simulink model "Model"  (R2021b)
settings: Solver=FixedStepAuto  StartTime=0.0  StopTime=simulation_time  FixedStep=0.02  RelTol=1e-3
values from neighbouring files (symbols this model uses):
  Cfx = 0.08268    [QuadStateSpaceModel.m]
  controller_flag = 1    [Simulation.m]
  d = 0.21    [QuadStateSpaceModel.m]
  g = 9.81    [QuadStateSpaceModel.m]
  Ix = 0.01    [QuadStateSpaceModel.m]
  Iy = 0.01    [QuadStateSpaceModel.m]
  Iz = 0.02    [QuadStateSpaceModel.m]
  Khover = correction(Khover)    [QuadStateSpaceModel.m]
  m = 1    [QuadStateSpaceModel.m]
  rho = 1.1840    (= 1.184)    [QuadStateSpaceModel.m]
libraries: sharedtransform x2, uavutilslib x2, shared6dof x2, aerolibasang x2, slpidlib x1
settings Model: Creator=siaem  LastModifiedBy=siaem
settings SolverCC: AlgebraicLoopSolver=TrustRegion
settings DataIOCC: ReturnWorkspaceOutputs=off
settings OptimizationCC: DefaultParameterBehavior=Inlined  EnhancedBackFolding=on  PassReuseOutputArgsAs=Individual arguments  ZeroExternalMemoryAtStartup=off  ZeroInternalMemoryAtStartup=off  MaxStackSize=64  OptimizeBlockOrder=speed  DifferentSizesBufferReuse=on  OptimizationCustomize=off  EfficientTunableParamExpr=on
settings DebuggingCC: ParameterTunabilityLossMsg=error  SFMachineParentedDataDiag=warning  ArithmeticOperatorsInVariantConditions=warning
settings HardwareCC: ProdBitPerPointer=32  ProdBitPerSizeT=32  ProdBitPerPtrDiffT=32  ProdLargestAtomicFloat=None  ProdIntDivRoundTo=Undefined  ProdEndianess=Unspecified  ProdWordSize=32  ProdHWDeviceType=Generic->Unspecified (assume 32-bit Generic)
settings SFSimCC: MATLABDynamicMemAlloc=off  CustomCodeUndefinedFunction=UseInterfaceOnly
settings RTWCC: Description=Embedded Coder  SystemTargetFile=ert.tlc  TemplateMakefile=ert_default_tmf  Toolchain=Catkin
settings CodeAppCC: ForceParamTrailComments=on  IgnoreCustomStorageClasses=off  OperatorAnnotations=on  SimulinkDataObjDesc=on  SFDataObjDesc=on  InsertBlockDesc=on
settings ERTTargetCC: ERTCustomFileTemplate=example_file_process.tlc

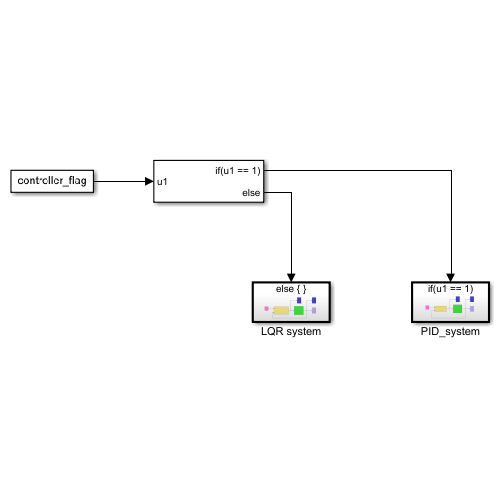
[thumbnail: Simulink's stored preview of the top-level diagram]
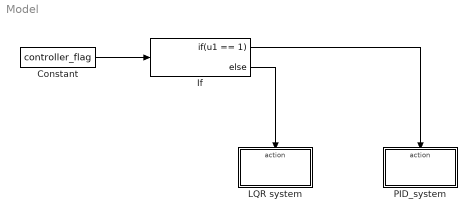
== system Model ==
  Constant : Constant  Value=controller_flag
  If : If  IfExpression=u1 == 1
  LQR system : Subsystem  TreatAsAtomicUnit=on
  PID_system : Subsystem  TreatAsAtomicUnit=on
  wires:
  Constant/1 -> If/1
  If/1 -> PID_system/Action
  If/2 -> LQR system/Action

== system Model/LQR system ==
  Action Port : ActionPort  ActionPortLabel=else
  Animation : Subsystem  Commented=on
  Controller : Subsystem
  Force & Moment Visualizer : Subsystem
  Setpoint : Subsystem
  States Visualizer : Subsystem
  quadrotor dynamic model : Subsystem
  wires:
  Controller/1(Forces/Moments) -> quadrotor dynamic model/1(Actuators), Force & Moment Visualizer/1(input)
  quadrotor dynamic model/1(States) -> Controller/2(States), Animation/1(In1), States Visualizer/1(output)
  Setpoint/1(Out1) -> Controller/1(setpoint)

== system Model/PID_system ==
  Action Port : ActionPort  ActionPortLabel=if(u1 == 1)
  Animation : Subsystem  Commented=on
  Controller : Subsystem
  Force & Moment Visualizer : Subsystem
  Setpoint : Subsystem
  States Visualizer : Subsystem
  quadrotor dynamic model : Subsystem
  wires:
  Setpoint/1(Out1) -> Controller/1(Setpoint)
  Controller/1(Forces Moments) -> quadrotor dynamic model/1(Actuators), Force & Moment Visualizer/1(input)
  quadrotor dynamic model/1(States) -> Animation/1(In1), States Visualizer/1(output), Controller/2(states)

== system Model/LQR system/Animation ==
  In1 : Inport
  Bus Selector : BusSelector  OutputSignals=X_e,attitude
  Rotation Angles to Quaternions : sharedtransform/Rotation Angles to Quaternions  rotationOrder=XYZ  aMode=aMode
      settings: SourceProductBaseCode=AE,PW,DR,MT,UV,VE
  UAV Animation : uavutilslib/UAV Animation  UAVType=Multirotor  UAVSize=1  InertialZDirection=Down  SampleTime=-1
      settings: SourceProductBaseCode=UV
  wires:
  Bus Selector/2 -> Rotation Angles to Quaternions/1  "<attitude>"
  Bus Selector/1 -> UAV Animation/1  "<X_e>"
  Rotation Angles to Quaternions/1 -> UAV Animation/2
  In1/1 -> Bus Selector/1

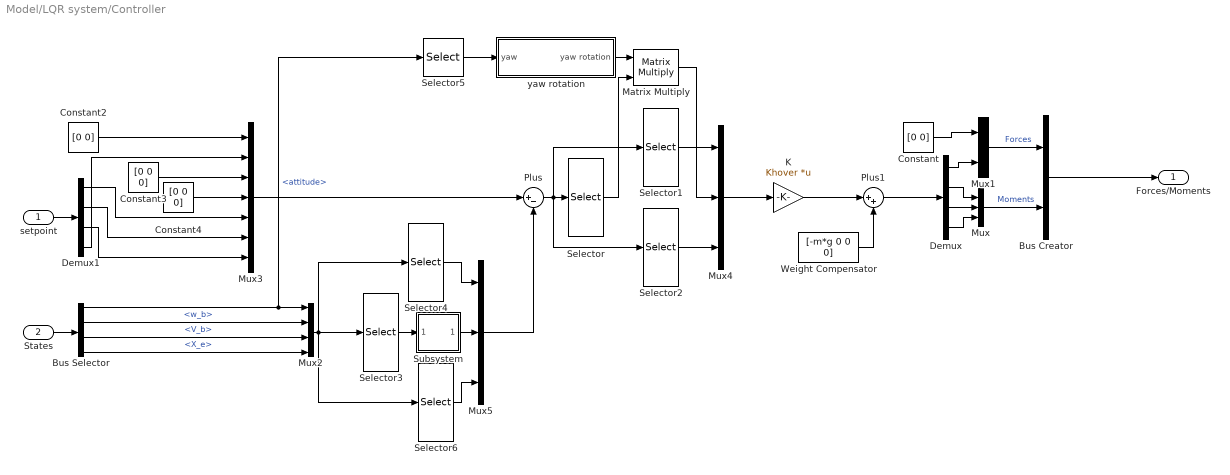
== system Model/LQR system/Controller ==
  setpoint : Inport
  States : Inport  Port=2
  Bus Creator : BusCreator  Inputs=2
  Bus Selector : BusSelector  OutputSignals=attitude,w_b,V_b,X_e
  Constant : Constant  Value=[0 0]
  Constant2 : Constant  Value=[0 0]
  Constant3 : Constant  Value=[0 0 0]
  Constant4 : Constant  Value=[0 0 0]
  Demux : Demux
  Demux1 : Demux
  K : Gain  Gain=Khover  Multiplication=Matrix(K*u) (u vector)
  Matrix Multiply : Product  Multiplication=Matrix(*)
  Mux : Mux  Inputs=3
  Mux1 : Mux  Inputs=2
  Mux2 : Mux
  Mux3 : Mux  Inputs=7
  Mux4 : Mux  Inputs=3
  Mux5 : Mux  Inputs=3
  Plus : Sum  Inputs=|+-
  Plus1 : Sum  Inputs=|++
  Selector : Selector  InputPortWidth=12  IndexOptions=Index vector (dialog)  Indices=[10 11]  OutputSizes=1
  Selector1 : Selector  InputPortWidth=12  IndexOptions=Index vector (dialog)  Indices=[1:9]  OutputSizes=1
  Selector2 : Selector  InputPortWidth=12  IndexOptions=Index vector (dialog)  Indices=12  OutputSizes=1
  Selector3 : Selector  InputPortWidth=12  IndexOptions=Index vector (dialog)  Indices=3  OutputSizes=1
  Selector4 : Selector  InputPortWidth=12  IndexOptions=Index vector (dialog)  Indices=[1,2]  OutputSizes=1
  Selector5 : Selector  InputPortWidth=3  IndexOptions=Index vector (dialog)  Indices=3  OutputSizes=1
  Selector6 : Selector  InputPortWidth=12  IndexOptions=Index vector (dialog)  Indices=[4:12]  OutputSizes=1
  Subsystem : Subsystem
  Weight Compensator : Constant  Value=[-m*g 0 0 0]
  yaw rotation : Subsystem
  Forces/Moments : Outport  VectorParamsAs1DForOutWhenUnconnected=off
  wires:
  Plus/1 -> Selector2/1, Selector1/1, Selector/1
  K/1 -> Plus1/1
  Weight Compensator/1 -> Plus1/2
  Plus1/1 -> Demux/1
  Demux/2 -> Mux/1
  Demux/3 -> Mux/2
  Demux/4 -> Mux/3
  Bus Creator/1 -> Forces/Moments/1
  Mux/1 -> Bus Creator/2  "Moments"
  Demux/1 -> Mux1/2
  Constant/1 -> Mux1/1
  Mux1/1 -> Bus Creator/1  "Forces"
  States/1 -> Bus Selector/1
  Bus Selector/1 -> Mux2/1, Selector5/1  "<attitude>"
  Bus Selector/2 -> Mux2/2  "<w_b>"
  Bus Selector/3 -> Mux2/3  "<V_b>"
  Bus Selector/4 -> Mux2/4  "<X_e>"
  setpoint/1 -> Demux1/1
  Demux1/4 -> Mux3/2
  Demux1/1 -> Mux3/5
  Demux1/2 -> Mux3/6
  Demux1/3 -> Mux3/7
  Constant2/1 -> Mux3/1
  Constant3/1 -> Mux3/3
  Constant4/1 -> Mux3/4
  Mux3/1 -> Plus/1
  Selector5/1 -> yaw rotation/1(yaw)
  yaw rotation/1(yaw rotation) -> Matrix Multiply/1
  Selector/1 -> Matrix Multiply/2
  Matrix Multiply/1 -> Mux4/2
  Selector1/1 -> Mux4/1
  Mux4/1 -> K/1
  Selector2/1 -> Mux4/3
  Mux2/1 -> Selector6/1, Selector4/1, Selector3/1
  Selector3/1 -> Subsystem/1(In1)
  Subsystem/1(Out1) -> Mux5/2
  Selector4/1 -> Mux5/1
  Selector6/1 -> Mux5/3
  Mux5/1 -> Plus/2

== system Model/LQR system/Force & Moment Visualizer ==
  input : Inport
  Demux3 : Demux
  Gain : Gain  Gain=-1
  Scope3 : Scope  NumInputPorts=4
  Selector : Selector  InputPortWidth=6  IndexOptions=Index vector (dialog)  Indices=[3, 4, 5, 6]  OutputSizes=1
  wires:
  Selector/1 -> Demux3/1
  Demux3/2 -> Scope3/2  "Tx"
  input/1 -> Selector/1
  Demux3/4 -> Scope3/4  "Tz"
  Demux3/3 -> Scope3/3  "Ty"
  Demux3/1 -> Gain/1  "Ft"
  Gain/1 -> Scope3/1

== system Model/LQR system/Setpoint ==
  From Workspace : FromWorkspace  VariableName=setpoint
  Out1 : Outport  VectorParamsAs1DForOutWhenUnconnected=off
  wires:
  From Workspace/1 -> Out1/1

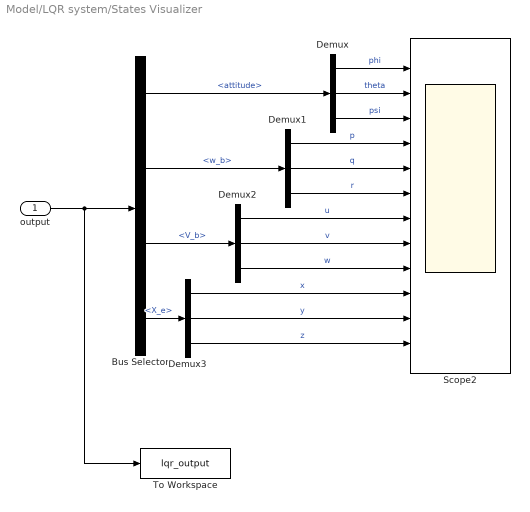
== system Model/LQR system/States Visualizer ==
  output : Inport
  Bus Selector : BusSelector  OutputSignals=attitude,w_b,V_b,X_e
  Demux{,1..3} (4 alike) : Demux  Outputs=3
  Scope2 : Scope  NumInputPorts=12
  To Workspace : ToWorkspace  VariableName=lqr_output  SaveFormat=Timeseries  SampleTime=-1
  wires:
  Demux1/3 -> Scope2/6  "r"
  Demux2/3 -> Scope2/9  "w"
  Demux2/1 -> Scope2/7  "u"
  Demux/2 -> Scope2/2  "theta"
  Demux/1 -> Scope2/1  "phi"
  Demux1/1 -> Scope2/4  "p"
  Demux1/2 -> Scope2/5  "q"
  Demux2/2 -> Scope2/8  "v"
  Demux3/1 -> Scope2/10  "x"
  Demux3/3 -> Scope2/12  "z"
  Demux/3 -> Scope2/3  "psi"
  Demux3/2 -> Scope2/11  "y"
  output/1 -> To Workspace/1, Bus Selector/1
  Bus Selector/1 -> Demux/1  "<attitude>"
  Bus Selector/2 -> Demux1/1  "<w_b>"
  Bus Selector/3 -> Demux2/1  "<V_b>"
  Bus Selector/4 -> Demux3/1  "<X_e>"

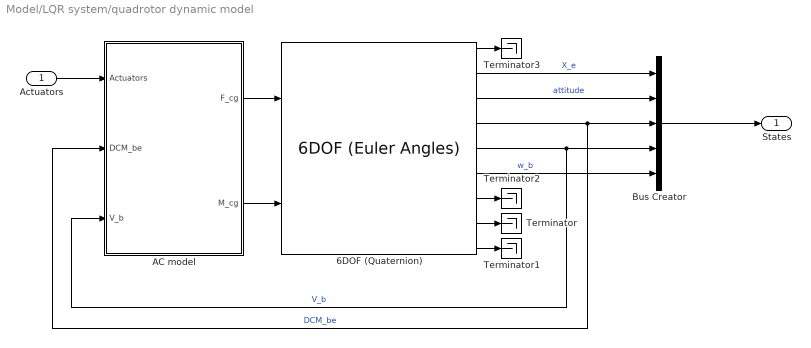
== system Model/LQR system/quadrotor dynamic model ==
  Actuators : Inport
  6DOF (Quaternion) : shared6dof/6DOF (Euler Angles)  units=Metric (MKS)  mtype=Fixed  rep=Euler Angles  xme_0=0  Vm_0=0  eul_0=0  pm_0=0  mass_0=m  mass_e=0.5  mass_f=2.0  inertia=[Ix,0,0;0,Iy,0;0,0,Iz]  inertia_e=eye(3)  inertia_f=2*eye(3)  k_quat=Vehicle.SixDOF.quatGain  vre_flag=on  abi_flag=on  aMode=aMode  xme_statename=''  Vm_statename=''  eul_statename=''  quat_statename=''  pm_statename=''  mass_statename=''
      settings: SourceProductBaseCode=AE,PW,DR,MT,UV,VE
  AC model : Subsystem
  Bus Creator : BusCreator  Inputs=5
  Terminator{,1..3} (4 alike) : Terminator
  States : Outport  VectorParamsAs1DForOutWhenUnconnected=off
  wires:
  6DOF (Quaternion)/9 -> Terminator1/1
  6DOF (Quaternion)/8 -> Terminator/1
  6DOF (Quaternion)/7 -> Terminator2/1
  Actuators/1 -> AC model/1(Actuators)
  6DOF (Quaternion)/1 -> Terminator3/1
  AC model/2(M_cg) -> 6DOF (Quaternion)/2
  AC model/1(F_cg) -> 6DOF (Quaternion)/1
  6DOF (Quaternion)/2 -> Bus Creator/1  "X_e"
  6DOF (Quaternion)/3 -> Bus Creator/2  "attitude"
  6DOF (Quaternion)/4 -> AC model/2(DCM_be), Bus Creator/3  "DCM_be"
  6DOF (Quaternion)/5 -> Bus Creator/4, AC model/3(V_b)  "V_b"
  6DOF (Quaternion)/6 -> Bus Creator/5  "w_b"
  Bus Creator/1 -> States/1

== system Model/PID_system/Animation ==
  In1 : Inport
  Bus Selector : BusSelector  OutputSignals=X_e,attitude
  Rotation Angles to Quaternions : sharedtransform/Rotation Angles to Quaternions  rotationOrder=XYZ  aMode=aMode
      settings: SourceProductBaseCode=AE,PW,DR,MT,UV,VE
  UAV Animation : uavutilslib/UAV Animation  UAVType=Multirotor  UAVSize=1  InertialZDirection=Down  SampleTime=-1
      settings: SourceProductBaseCode=UV
  wires:
  Bus Selector/2 -> Rotation Angles to Quaternions/1  "<attitude>"
  Bus Selector/1 -> UAV Animation/1  "<X_e>"
  Rotation Angles to Quaternions/1 -> UAV Animation/2
  In1/1 -> Bus Selector/1

== system Model/PID_system/Controller ==
  Setpoint : Inport
  states : Inport  Port=2
  Bus Creator : BusCreator  Inputs=2
  Position Controller : Subsystem
  Roll/Pitch Controller : Subsystem
  Setpoint1 : InportShadow
  Yaw Controller : Subsystem
  Forces Moments : Outport
  wires:
  Roll/Pitch Controller/1(Moments) -> Bus Creator/2  "Moments"
  Position Controller/1(Thrust) -> Bus Creator/1  "Forces"
  Setpoint/1 -> Position Controller/1(Desired Position)
  Position Controller/2(Desired Roll/Pitch) -> Roll/Pitch Controller/1(Desired Roll/Pitch)
  Bus Creator/1 -> Forces Moments/1
  states/1 -> Roll/Pitch Controller/3(Estimated Roll/Pitch), Position Controller/2(Estimated Position), Yaw Controller/1(yaw)
  Yaw Controller/1(tau_yaw) -> Roll/Pitch Controller/2(tau_yaw)
  Setpoint1/1 -> Yaw Controller/2(setpoint)

== system Model/PID_system/Force & Moment Visualizer ==
  input : Inport
  Demux3 : Demux
  Gain : Gain  Gain=-1
  Scope3 : Scope  NumInputPorts=4
  Selector : Selector  InputPortWidth=6  IndexOptions=Index vector (dialog)  Indices=[3, 4, 5, 6]  OutputSizes=1
  wires:
  Selector/1 -> Demux3/1
  Demux3/2 -> Scope3/2  "Tx"
  input/1 -> Selector/1
  Demux3/4 -> Scope3/4  "Tz"
  Demux3/3 -> Scope3/3  "Ty"
  Demux3/1 -> Gain/1  "Ft"
  Gain/1 -> Scope3/1

== system Model/PID_system/Setpoint ==
  From Workspace : FromWorkspace  VariableName=setpoint
  Out1 : Outport  VectorParamsAs1DForOutWhenUnconnected=off
  wires:
  From Workspace/1 -> Out1/1

== system Model/PID_system/States Visualizer ==
  output : Inport
  Bus Selector : BusSelector  OutputSignals=attitude,w_b,V_b,X_e
  Demux{,1..3} (4 alike) : Demux  Outputs=3
  Scope2 : Scope  NumInputPorts=12
  To Workspace : ToWorkspace  VariableName=pid_output  SaveFormat=Timeseries  SampleTime=-1
  wires:
  Demux1/3 -> Scope2/6  "r"
  Demux2/3 -> Scope2/9  "w"
  Demux2/1 -> Scope2/7  "u"
  Demux/2 -> Scope2/2  "theta"
  Demux/1 -> Scope2/1  "phi"
  Demux1/1 -> Scope2/4  "p"
  Demux1/2 -> Scope2/5  "q"
  Demux2/2 -> Scope2/8  "v"
  Demux3/1 -> Scope2/10  "x"
  Demux3/3 -> Scope2/12  "z"
  Demux/3 -> Scope2/3  "psi"
  Demux3/2 -> Scope2/11  "y"
  output/1 -> To Workspace/1, Bus Selector/1
  Bus Selector/1 -> Demux/1  "<attitude>"
  Bus Selector/2 -> Demux1/1  "<w_b>"
  Bus Selector/3 -> Demux2/1  "<V_b>"
  Bus Selector/4 -> Demux3/1  "<X_e>"

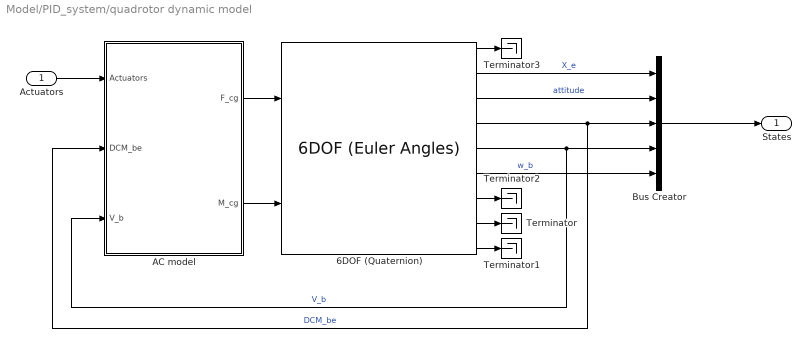
== system Model/PID_system/quadrotor dynamic model ==
  Actuators : Inport
  6DOF (Quaternion) : shared6dof/6DOF (Euler Angles)  units=Metric (MKS)  mtype=Fixed  rep=Euler Angles  xme_0=0  Vm_0=0  eul_0=0  pm_0=0  mass_0=m  mass_e=0.5  mass_f=2.0  inertia=[Ix,0,0;0,Iy,0;0,0,Iz]  inertia_e=eye(3)  inertia_f=2*eye(3)  k_quat=Vehicle.SixDOF.quatGain  vre_flag=on  abi_flag=on  aMode=aMode  xme_statename=''  Vm_statename=''  eul_statename=''  quat_statename=''  pm_statename=''  mass_statename=''
      settings: SourceProductBaseCode=AE,PW,DR,MT,UV,VE
  AC model : Subsystem
  Bus Creator : BusCreator  Inputs=5
  Terminator{,1..3} (4 alike) : Terminator
  States : Outport  VectorParamsAs1DForOutWhenUnconnected=off
  wires:
  6DOF (Quaternion)/9 -> Terminator1/1
  6DOF (Quaternion)/8 -> Terminator/1
  6DOF (Quaternion)/7 -> Terminator2/1
  Actuators/1 -> AC model/1(Actuators)
  6DOF (Quaternion)/1 -> Terminator3/1
  AC model/2(M_cg) -> 6DOF (Quaternion)/2
  AC model/1(F_cg) -> 6DOF (Quaternion)/1
  6DOF (Quaternion)/2 -> Bus Creator/1  "X_e"
  6DOF (Quaternion)/3 -> Bus Creator/2  "attitude"
  6DOF (Quaternion)/4 -> AC model/2(DCM_be), Bus Creator/3  "DCM_be"
  6DOF (Quaternion)/5 -> Bus Creator/4, AC model/3(V_b)  "V_b"
  6DOF (Quaternion)/6 -> Bus Creator/5  "w_b"
  Bus Creator/1 -> States/1

== system Model/LQR system/Controller/Subsystem ==
  In1 : Inport
  If : If  IfExpression=u1 > 3.139 | u1 < 0
  If Action Subsystem : Subsystem  TreatAsAtomicUnit=on
  If Action Subsystem1 : Subsystem  TreatAsAtomicUnit=on
  Merge : Merge
  Out1 : Outport
  wires:
  If/1 -> If Action Subsystem/Action
  In1/1 -> If Action Subsystem1/1(In1), If Action Subsystem/1(In1), If/1
  If Action Subsystem/1(Out1) -> Merge/1
  If Action Subsystem1/1(Out1) -> Merge/2
  If/2 -> If Action Subsystem1/Action
  Merge/1 -> Out1/1

== system Model/LQR system/Controller/yaw rotation ==
  yaw : Inport
  Gain1 : Gain  Gain=-1
  Matrix Concatenate : Concatenate  Mode=Multidimensional array  ConcatenateDimension=2
  Trigonometric Function : Trigonometry  Operator=sincos
  Vector Concatenate : Concatenate
  Vector Concatenate1 : Concatenate
  yaw rotation : Outport
  wires:
  Trigonometric Function/1 -> Gain1/1, Vector Concatenate1/1
  Trigonometric Function/2 -> Vector Concatenate1/2, Vector Concatenate/1
  Vector Concatenate1/1 -> Matrix Concatenate/2
  Vector Concatenate/1 -> Matrix Concatenate/1
  Gain1/1 -> Vector Concatenate/2
  yaw/1 -> Trigonometric Function/1
  Matrix Concatenate/1 -> yaw rotation/1

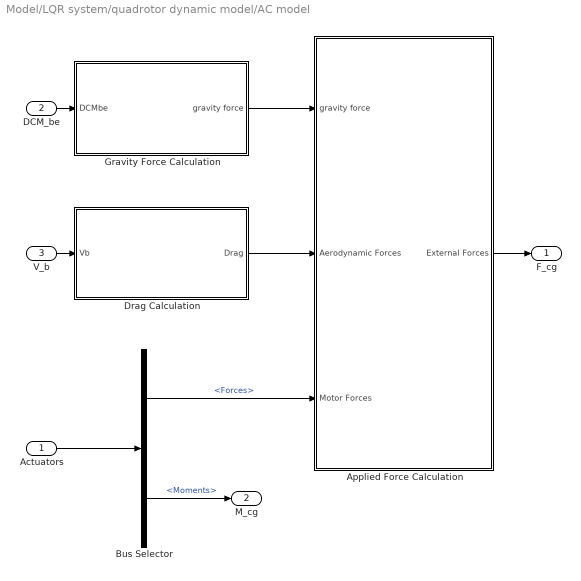
== system Model/LQR system/quadrotor dynamic model/AC model ==
  Actuators : Inport
  DCM_be : Inport  Port=2
  V_b : Inport  Port=3  Unit=m/s
  Applied Force Calculation : Subsystem
  Bus Selector : BusSelector  OutputSignals=Forces,Moments
  Drag Calculation : Subsystem
  Gravity Force Calculation : Subsystem
  F_cg : Outport  Unit=N  VectorParamsAs1DForOutWhenUnconnected=off
  M_cg : Outport  Port=2  Unit=N*m  VectorParamsAs1DForOutWhenUnconnected=off
  wires:
  Applied Force Calculation/1(External Forces) -> F_cg/1
  Actuators/1 -> Bus Selector/1
  Gravity Force Calculation/1(gravity force) -> Applied Force Calculation/1(gravity force)
  DCM_be/1 -> Gravity Force Calculation/1(DCMbe)
  V_b/1 -> Drag Calculation/1(Vb)
  Drag Calculation/1(Drag) -> Applied Force Calculation/2(Aerodynamic Forces)
  Bus Selector/1 -> Applied Force Calculation/3(Motor Forces)  "<Forces>"
  Bus Selector/2 -> M_cg/1  "<Moments>"

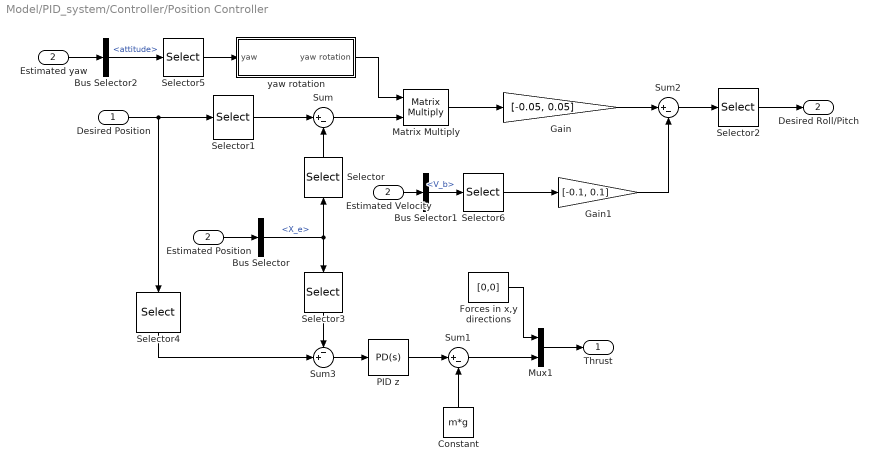
== system Model/PID_system/Controller/Position Controller ==
  Desired Position : Inport
  Estimated Position : Inport  Port=2
  Bus Selector : BusSelector  OutputSignals=X_e
  Bus Selector1 : BusSelector  OutputSignals=V_b
  Bus Selector2 : BusSelector  OutputSignals=attitude
  Constant : Constant  Value=m*g
  Estimated Velocity : InportShadow  Port=2
  Estimated yaw : InportShadow  Port=2
  Forces in x,y directions : Constant  Value=[0,0]
  Gain : Gain  Gain=[-0.05, 0.05]
  Gain1 : Gain  Gain=[-0.1, 0.1]
  Matrix Multiply : Product  Multiplication=Matrix(*)
  Mux1 : Mux  Inputs=2
  PID z : slpidlib/PID Controller  Controller=PD  Form=Parallel  TimeDomain=Continuous-time  UseExternalTs=off  SampleTime=-1  IntegratorMethod=Forward Euler  FilterMethod=Forward Euler  ControllerParametersSource=internal  P=4  I=0.0175763028202864  D=7  UseFilter=on  N=10  TunerSelectOption=Transfer Function Based (PID Tuner App)  InitialConditionSource=internal  InitialConditionForIntegrator=0  InitialConditionForFilter=0  DifferentiatorICPrevScaledInput=0  ExternalReset=none  TrackingMode=off  Kt=1  LimitOutput=off  SatLimitsSource=internal  UpperSaturationLimit=inf  LowerSaturationLimit=-inf  LinearizeAsGain=on  AntiWindupMode=none  Kb=1  POutMin=[]  POutMax=[]  IOutMin=[]  IOutMax=[]  DOutMin=[]  DOutMax=[]  NOutMin=[]  NOutMax=[]  SumOutMin=[]  SumOutMax=[]  SaturationOutMin=[]  SaturationOutMax=[]  PParamMin=[]  PParamMax=[]  IParamMin=[]  IParamMax=[]  DParamMin=[]  DParamMax=[]  NParamMin=[]  NParamMax=[]  KbParamMin=[]  KbParamMax=[]  KtParamMin=[]  KtParamMax=[]  KbOutMin=[]  KbOutMax=[]  KtOutMin=[]  KtOutMax=[]  IntegratorOutMin=[]  IntegratorOutMax=[]  FilterOutMin=[]  FilterOutMax=[]  SumI1OutMin=[]  SumI1OutMax=[]  SumI2OutMin=[]  SumI2OutMax=[]  SumI3OutMin=[]  SumI3OutMax=[]  SumI4OutMin=[]  SumI4OutMax=[]  SumDOutMin=[]  SumDOutMax=[]  DifferentiatorOutMin=[]  DifferentiatorOutMax=[]  FilterDiffOutCoefMin=[]  FilterDiffOutCoefMax=[]  ReciprocalOutMin=[]  ReciprocalOutMax=[]  SumDenOutMin=[]  SumDenOutMax=[]  SumNumOutMin=[]  SumNumOutMax=[]  DivideOutMin=[]  DivideOutMax=[]  UdiffTsProdOutMin=[]  UdiffTsProdOutMax=[]  NTsProdOutMin=[]  NTsProdOutMax=[]  UintegralTsProdOutMin=[]  UintegralTsProdOutMax=[]  UngainTsProdOutMin=[]  UngainTsProdOutMax=[]  IntegratorContinuousStateAttributes=''  IntegratorStateMustResolveToSignalObject=off  IntegratorRTWStateStorageClass=Auto  FilterContinuousStateAttributes=''  FilterStateMustResolveToSignalObject=off  FilterRTWStateStorageClass=Auto  ParallelPVariant=InternalParameters  IdealPVariant=Disabled  IVariant=Disabled  DVariant=InternalParameters  IntegratorVariant=Disabled  SatVariant=Disabled  AWVariant=Disabled  PCopyVariant=Disabled  TRVariant=Disabled  FdbkBlocksVariant=Forward  IdealPFdbkVariant=Disabled  SatFdbkVariant=Disabled  DerivativeFilterVariant=ContFilter  NVariant=InternalParameters  NCopyVariant=Disabled  FilterICVariant=InternalICsFilter  IntegratorICVariant=Disabled  ExternalResetVariant=Disabled  TRSumVariant=Passthrough  SumFdbkVariant=Disabled  SumVariant=Sum_PD  TsampFilterVariant=InternalTs  TsampNgainVariant=Passthrough  TsampIntegralVariant=Disabled_SignalSpec  ExternalSaturationOutDataTypeStr=Inherit: Same as second input
  Selector : Selector  InputPortWidth=3  IndexOptions=Index vector (dialog)  Indices=[1 2]  OutputSizes=1
  Selector1 : Selector  InputPortWidth=4  IndexOptions=Index vector (dialog)  Indices=[1 2]  OutputSizes=1
  Selector2 : Selector  InputPortWidth=2  IndexOptions=Index vector (dialog)  Indices=[2 1]  OutputSizes=1
  Selector3 : Selector  InputPortWidth=3  IndexOptions=Index vector (dialog)  Indices=3  OutputSizes=1
  Selector4 : Selector  InputPortWidth=4  IndexOptions=Index vector (dialog)  Indices=3  OutputSizes=1
  Selector5 : Selector  InputPortWidth=3  IndexOptions=Index vector (dialog)  Indices=3  OutputSizes=1
  Selector6 : Selector  InputPortWidth=3  IndexOptions=Index vector (dialog)  Indices=[1 2]  OutputSizes=1
  Sum : Sum  Inputs=|+-
  Sum1 : Sum  Inputs=|+-
  Sum2 : Sum  Inputs=|+-
  Sum3 : Sum  Inputs=-+|
  yaw rotation : Subsystem
  Thrust : Outport  VectorParamsAs1DForOutWhenUnconnected=off
  Desired Roll/Pitch : Outport  Port=2  VectorParamsAs1DForOutWhenUnconnected=off
  wires:
  Selector/1 -> Sum/2
  Desired Position/1 -> Selector1/1, Selector4/1
  Selector1/1 -> Sum/1
  Constant/1 -> Sum1/2
  Mux1/1 -> Thrust/1
  Sum1/1 -> Mux1/2
  Forces in x,y directions/1 -> Mux1/1
  Selector3/1 -> Sum3/1
  Selector4/1 -> Sum3/2
  PID z/1 -> Sum1/1
  Sum3/1 -> PID z/1
  Selector5/1 -> yaw rotation/1(yaw)
  Sum/1 -> Matrix Multiply/2
  yaw rotation/1(yaw rotation) -> Matrix Multiply/1
  Estimated Position/1 -> Bus Selector/1
  Bus Selector/1 -> Selector3/1, Selector/1  "<X_e>"
  Estimated yaw/1 -> Bus Selector2/1
  Bus Selector2/1 -> Selector5/1  "<attitude>"
  Matrix Multiply/1 -> Gain/1
  Selector6/1 -> Gain1/1
  Gain1/1 -> Sum2/2
  Sum2/1 -> Selector2/1
  Selector2/1 -> Desired Roll/Pitch/1
  Gain/1 -> Sum2/1
  Estimated Velocity/1 -> Bus Selector1/1
  Bus Selector1/1 -> Selector6/1  "<V_b>"

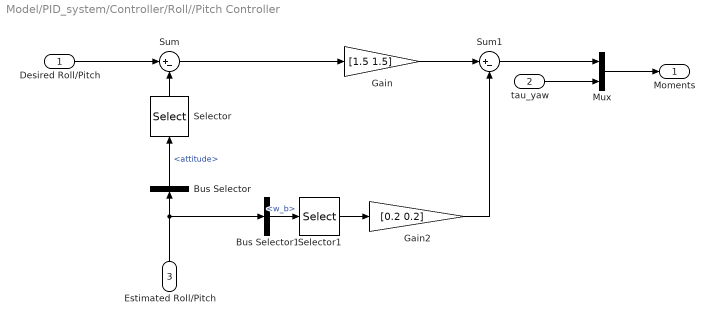
== system Model/PID_system/Controller/Roll//Pitch Controller ==
  Desired Roll/Pitch : Inport
  tau_yaw : Inport  Port=2
  Estimated Roll/Pitch : Inport  Port=3
  Bus Selector : BusSelector  OutputSignals=attitude
  Bus Selector1 : BusSelector  OutputSignals=w_b
  Gain : Gain  Gain=[1.5 1.5]
  Gain2 : Gain  Gain=[0.2 0.2]
  Mux : Mux  Inputs=2
  Selector : Selector  InputPortWidth=3  IndexOptions=Index vector (dialog)  Indices=[1 2]  OutputSizes=1
  Selector1 : Selector  InputPortWidth=3  IndexOptions=Index vector (dialog)  Indices=[1 2]  OutputSizes=1
  Sum : Sum  Inputs=|+-
  Sum1 : Sum  Inputs=|+-
  Moments : Outport  VectorParamsAs1DForOutWhenUnconnected=off
  wires:
  Desired Roll/Pitch/1 -> Sum/1
  Mux/1 -> Moments/1
  Sum/1 -> Gain/1
  tau_yaw/1 -> Mux/2
  Estimated Roll/Pitch/1 -> Bus Selector1/1, Bus Selector/1
  Selector/1 -> Sum/2
  Bus Selector/1 -> Selector/1  "<attitude>"
  Bus Selector1/1 -> Selector1/1  "<w_b>"
  Selector1/1 -> Gain2/1
  Gain/1 -> Sum1/1
  Gain2/1 -> Sum1/2
  Sum1/1 -> Mux/1

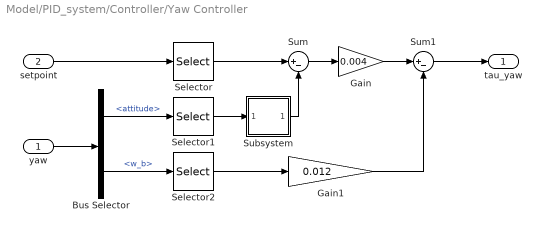
== system Model/PID_system/Controller/Yaw Controller ==
  yaw : Inport
  setpoint : Inport  Port=2
  Bus Selector : BusSelector  OutputSignals=attitude,w_b
  Gain : Gain  Gain=0.004
  Gain1 : Gain  Gain=0.012
  Selector : Selector  InputPortWidth=4  IndexOptions=Index vector (dialog)  Indices=4  OutputSizes=1
  Selector1 : Selector  InputPortWidth=3  IndexOptions=Index vector (dialog)  Indices=3  OutputSizes=1
  Selector2 : Selector  InputPortWidth=3  IndexOptions=Index vector (dialog)  Indices=3  OutputSizes=1
  Subsystem : Subsystem
  Sum : Sum  Inputs=|+-
  Sum1 : Sum  Inputs=|+-
  tau_yaw : Outport
  wires:
  setpoint/1 -> Selector/1
  yaw/1 -> Bus Selector/1
  Bus Selector/2 -> Selector2/1  "<w_b>"
  Sum/1 -> Gain/1
  Gain/1 -> Sum1/1
  Sum1/1 -> tau_yaw/1
  Selector2/1 -> Gain1/1
  Gain1/1 -> Sum1/2
  Selector/1 -> Sum/1
  Bus Selector/1 -> Selector1/1  "<attitude>"
  Selector1/1 -> Subsystem/1(In1)
  Subsystem/1(Out1) -> Sum/2

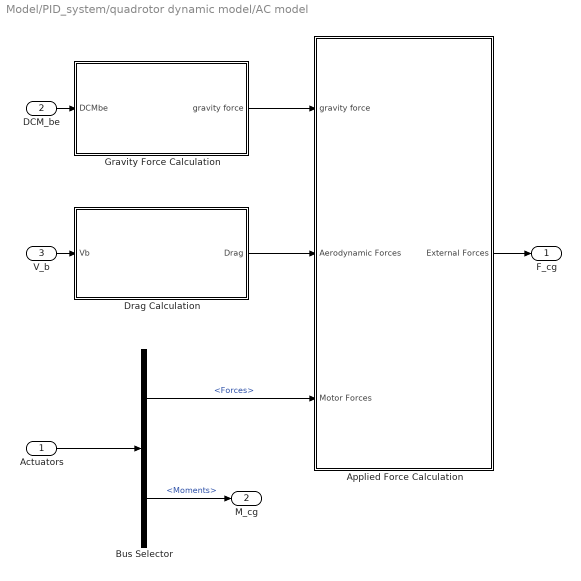
== system Model/PID_system/quadrotor dynamic model/AC model ==
  Actuators : Inport
  DCM_be : Inport  Port=2
  V_b : Inport  Port=3  Unit=m/s
  Applied Force Calculation : Subsystem
  Bus Selector : BusSelector  OutputSignals=Forces,Moments
  Drag Calculation : Subsystem
  Gravity Force Calculation : Subsystem
  F_cg : Outport  Unit=N  VectorParamsAs1DForOutWhenUnconnected=off
  M_cg : Outport  Port=2  Unit=N*m  VectorParamsAs1DForOutWhenUnconnected=off
  wires:
  Applied Force Calculation/1(External Forces) -> F_cg/1
  Actuators/1 -> Bus Selector/1
  Gravity Force Calculation/1(gravity force) -> Applied Force Calculation/1(gravity force)
  DCM_be/1 -> Gravity Force Calculation/1(DCMbe)
  V_b/1 -> Drag Calculation/1(Vb)
  Drag Calculation/1(Drag) -> Applied Force Calculation/2(Aerodynamic Forces)
  Bus Selector/1 -> Applied Force Calculation/3(Motor Forces)  "<Forces>"
  Bus Selector/2 -> M_cg/1  "<Moments>"

== system Model/LQR system/Controller/Subsystem/If Action Subsystem ==
  In1 : Inport
  Action Port : ActionPort  ActionPortLabel=if(u1 > 3.139 | u1 < 0)
  Constant : Constant  Value=2*pi
  Plus : Sum
  Out1 : Outport
  wires:
  Constant/1 -> Plus/1
  In1/1 -> Plus/2
  Plus/1 -> Out1/1

== system Model/LQR system/Controller/Subsystem/If Action Subsystem1 ==
  In1 : Inport
  Action Port : ActionPort  ActionPortLabel=else
  Out1 : Outport
  wires:
  In1/1 -> Out1/1

== system Model/LQR system/quadrotor dynamic model/AC model/Applied Force Calculation ==
  gravity force : Inport  Unit=N
  Aerodynamic Forces : Inport  Port=2  Unit=N
  Motor Forces : Inport  Port=3  Unit=N
  Add1 : Sum  Inputs=+++
  Signal Specification : SignalSpecification  Dimensions=3
  External Forces : Outport  Unit=N  VectorParamsAs1DForOutWhenUnconnected=off
  wires:
  Add1/1 -> Signal Specification/1
  Motor Forces/1 -> Add1/3  "Motor Thrust"
  Aerodynamic Forces/1 -> Add1/2
  gravity force/1 -> Add1/1
  Signal Specification/1 -> External Forces/1

== system Model/LQR system/quadrotor dynamic model/AC model/Drag Calculation ==
  Vb : Inport  Unit=m/second
  Constant : Constant  Value=rho
  Drag Calc : Subsystem
  Gain3 : Gain  Gain=-1
  Product : Product  RndMeth=Zero
  Sign : Signum  ZeroCross=off
  Drag : Outport  Unit=N  VectorParamsAs1DForOutWhenUnconnected=off
  wires:
  Constant/1 -> Drag Calc/1(Density)
  Sign/1 -> Gain3/1
  Drag Calc/1(drag) -> Product/1
  Gain3/1 -> Product/2
  Product/1 -> Drag/1  "xDrag"
  Vb/1 -> Sign/1, Drag Calc/2(vel)

== system Model/LQR system/quadrotor dynamic model/AC model/Gravity Force Calculation ==
  DCMbe : Inport
  Constant : Constant  Value=[0, 0, g]
  Gain1 : Gain  Gain=m
  Product : Product  Multiplication=Matrix(*)
  gravity force : Outport  Unit=N  VectorParamsAs1DForOutWhenUnconnected=off
  wires:
  Constant/1 -> Gain1/1
  Gain1/1 -> Product/2  "gravity force NED"
  Product/1 -> gravity force/1
  DCMbe/1 -> Product/1

== system Model/PID_system/Controller/Position Controller/yaw rotation ==
  yaw : Inport
  Gain1 : Gain  Gain=-1
  Matrix Concatenate : Concatenate  Mode=Multidimensional array  ConcatenateDimension=2
  Trigonometric Function : Trigonometry  Operator=sincos
  Vector Concatenate : Concatenate
  Vector Concatenate1 : Concatenate
  yaw rotation : Outport
  wires:
  Trigonometric Function/1 -> Gain1/1, Vector Concatenate1/1
  Trigonometric Function/2 -> Vector Concatenate1/2, Vector Concatenate/1
  Vector Concatenate1/1 -> Matrix Concatenate/2
  Vector Concatenate/1 -> Matrix Concatenate/1
  Gain1/1 -> Vector Concatenate/2
  yaw/1 -> Trigonometric Function/1
  Matrix Concatenate/1 -> yaw rotation/1

== system Model/PID_system/Controller/Yaw Controller/Subsystem ==
  In1 : Inport
  If : If  IfExpression=u1 > 3.139 | u1 < 0
  If Action Subsystem : Subsystem  TreatAsAtomicUnit=on
  If Action Subsystem1 : Subsystem  TreatAsAtomicUnit=on
  Merge : Merge
  Out1 : Outport
  wires:
  If/1 -> If Action Subsystem/Action
  In1/1 -> If Action Subsystem1/1(In1), If Action Subsystem/1(In1), If/1
  If Action Subsystem/1(Out1) -> Merge/1
  If Action Subsystem1/1(Out1) -> Merge/2
  If/2 -> If Action Subsystem1/Action
  Merge/1 -> Out1/1

== system Model/PID_system/quadrotor dynamic model/AC model/Applied Force Calculation ==
  gravity force : Inport  Unit=N
  Aerodynamic Forces : Inport  Port=2  Unit=N
  Motor Forces : Inport  Port=3  Unit=N
  Add1 : Sum  Inputs=+++
  Signal Specification : SignalSpecification  Dimensions=3
  External Forces : Outport  Unit=N  VectorParamsAs1DForOutWhenUnconnected=off
  wires:
  Add1/1 -> Signal Specification/1
  Motor Forces/1 -> Add1/3  "Motor Thrust"
  Aerodynamic Forces/1 -> Add1/2
  gravity force/1 -> Add1/1
  Signal Specification/1 -> External Forces/1

== system Model/PID_system/quadrotor dynamic model/AC model/Drag Calculation ==
  Vb : Inport  Unit=m/second
  Constant : Constant  Value=rho
  Drag Calc : Subsystem
  Gain3 : Gain  Gain=-1
  Product : Product  RndMeth=Zero
  Sign : Signum  ZeroCross=off
  Drag : Outport  Unit=N  VectorParamsAs1DForOutWhenUnconnected=off
  wires:
  Constant/1 -> Drag Calc/1(Density)
  Sign/1 -> Gain3/1
  Drag Calc/1(drag) -> Product/1
  Gain3/1 -> Product/2
  Product/1 -> Drag/1  "xDrag"
  Vb/1 -> Sign/1, Drag Calc/2(vel)

== system Model/PID_system/quadrotor dynamic model/AC model/Gravity Force Calculation ==
  DCMbe : Inport
  Constant : Constant  Value=[0, 0, g]
  Gain1 : Gain  Gain=m
  Product : Product  Multiplication=Matrix(*)
  gravity force : Outport  Unit=N  VectorParamsAs1DForOutWhenUnconnected=off
  wires:
  Constant/1 -> Gain1/1
  Gain1/1 -> Product/2  "gravity force NED"
  Product/1 -> gravity force/1
  DCMbe/1 -> Product/1

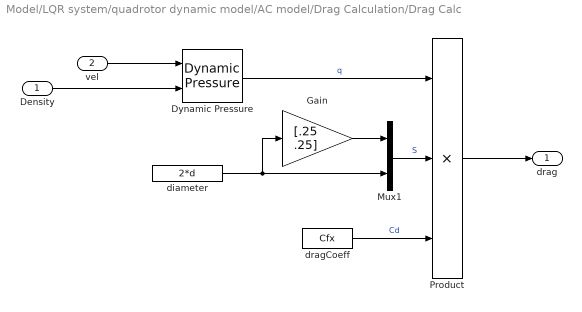
== system Model/LQR system/quadrotor dynamic model/AC model/Drag Calculation/Drag Calc ==
  Density : Inport  Unit=kg/m^3
  vel : Inport  Port=2  Unit=m/s
  Dynamic Pressure : aerolibasang/Dynamic Pressure
  Gain : Gain  Gain=[.25 .25]
  Mux1 : Mux  Inputs=2
  Product : Product  Inputs=3  RndMeth=Zero
  diameter : Constant  Value=2*d  SampleTime=0
  dragCoeff : Constant  Value=Cfx  SampleTime=0
  drag : Outport  Unit=N  VectorParamsAs1DForOutWhenUnconnected=off
  wires:
  Product/1 -> drag/1
  dragCoeff/1 -> Product/3  "Cd"
  Dynamic Pressure/1 -> Product/1  "q"
  diameter/1 -> Gain/1, Mux1/2
  Mux1/1 -> Product/2  "S"
  Gain/1 -> Mux1/1
  vel/1 -> Dynamic Pressure/1
  Density/1 -> Dynamic Pressure/2

== system Model/PID_system/Controller/Yaw Controller/Subsystem/If Action Subsystem ==
  In1 : Inport
  Action Port : ActionPort  ActionPortLabel=if(u1 > 3.139 | u1 < 0)
  Constant : Constant  Value=2*pi
  Plus : Sum
  Out1 : Outport
  wires:
  Constant/1 -> Plus/1
  In1/1 -> Plus/2
  Plus/1 -> Out1/1

== system Model/PID_system/Controller/Yaw Controller/Subsystem/If Action Subsystem1 ==
  In1 : Inport
  Action Port : ActionPort  ActionPortLabel=else
  Out1 : Outport
  wires:
  In1/1 -> Out1/1

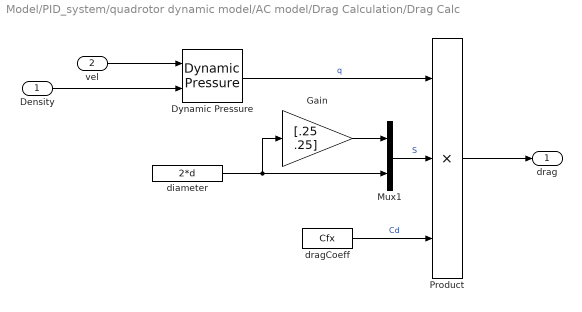
== system Model/PID_system/quadrotor dynamic model/AC model/Drag Calculation/Drag Calc ==
  Density : Inport  Unit=kg/m^3
  vel : Inport  Port=2  Unit=m/s
  Dynamic Pressure : aerolibasang/Dynamic Pressure
  Gain : Gain  Gain=[.25 .25]
  Mux1 : Mux  Inputs=2
  Product : Product  Inputs=3  RndMeth=Zero
  diameter : Constant  Value=2*d  SampleTime=0
  dragCoeff : Constant  Value=Cfx  SampleTime=0
  drag : Outport  Unit=N  VectorParamsAs1DForOutWhenUnconnected=off
  wires:
  Product/1 -> drag/1
  dragCoeff/1 -> Product/3  "Cd"
  Dynamic Pressure/1 -> Product/1  "q"
  diameter/1 -> Gain/1, Mux1/2
  Mux1/1 -> Product/2  "S"
  Gain/1 -> Mux1/1
  vel/1 -> Dynamic Pressure/1
  Density/1 -> Dynamic Pressure/2
